simulink model "seasat"  (Simulink 5.0)
settings: Solver=ode23s  StartTime=0.0  StopTime=6000  RelTol=1e-3
values from neighbouring files (symbols this model uses):
  A = sqrt(ri*rf/(1-cos(phi)))*sin(phi)    [lambert.m]
  B = 2/re    (= 3.13571041087e-07)    [atmosphere.m]    (also in kepler.m = cos(e)-(pi/2-e)*sin(e))
  K = liftddf(mach,CL,sweep,b^2/S)    [accelclimb.m]    (also in liftddf.m = S*K100+(1-S)*K0; maneuver.m)
libraries: simulink x1

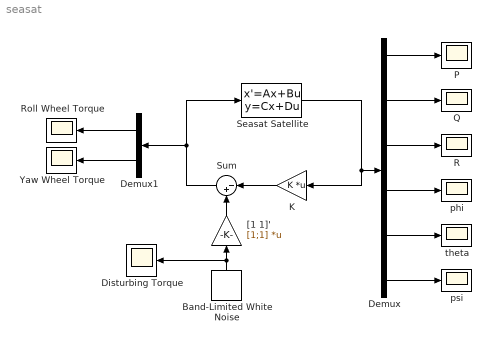
== system seasat ==
  Band-Limited White Noise : simulink/Sources/Band-Limited White Noise  Orientation=up  Cov=[1e-7]  Ts=0.1  seed=[23341]
  Demux : Demux  Outputs=6
  Demux1 : Demux  Orientation=left  Outputs=2
  Disturbing Torque : Scope
      settings: SaveName=dist  DataFormat=Array
  K : Gain  Orientation=left  Gain=K  Multiplication=Matrix(K*u)  SaturateOnIntegerOverflow=on
  P : Scope
      settings: SaveName=P  DataFormat=Array  Decimation=100
  Q : Scope
      settings: SaveName=Q  DataFormat=Array  Decimation=100
  R : Scope
      settings: SaveName=R  DataFormat=Array  Decimation=100
  Roll Wheel Torque : Scope
      settings: SaveName=u1  DataFormat=Array  Decimation=100
  Seasat Satellite : StateSpace  A=A  B=B  C=eye(size(A))  D=zeros(size(B))  X0=[0 0 0 0.01 0.002 0]'
  Sum : Sum  Orientation=left  Inputs=|-+  SaturateOnIntegerOverflow=on
  Yaw Wheel Torque : Scope
      settings: SaveName=u2  DataFormat=Array  Decimation=100
  "[1 1]'" : Gain  Orientation=up  Gain=[1;1]  Multiplication=Matrix(K*u)  SaturateOnIntegerOverflow=on
  phi : Scope
      settings: SaveName=phi  DataFormat=Array  Decimation=100
  psi : Scope
      settings: SaveName=psi  DataFormat=Array  Decimation=100
  theta : Scope
      settings: SaveName=theta  DataFormat=Array  Decimation=100
  wires:
  Seasat Satellite/1 -> K/1, Demux/1
  K/1 -> Sum/1
  Band-Limited White Noise/1 -> "[1 1]'"/1, Disturbing Torque/1
  "[1 1]'"/1 -> Sum/2
  Sum/1 -> Seasat Satellite/1, Demux1/1
  Demux/1 -> P/1
  Demux/2 -> Q/1
  Demux/3 -> R/1
  Demux/4 -> phi/1
  Demux/5 -> theta/1
  Demux/6 -> psi/1
  Demux1/2 -> Yaw Wheel Torque/1
  Demux1/1 -> Roll Wheel Torque/1
